simulink model "Dong_co_mot_chieu_KTSS"  (R2019a)
settings: Solver=VariableStepAuto  StartTime=0.0  StopTime=10.0  RelTol=1e-3
libraries: powerlib x5
settings Model: Creator=Admin  LastModifiedBy=Admin

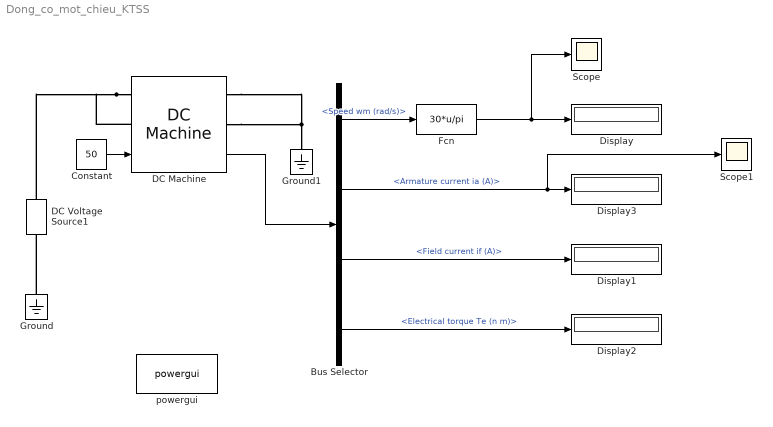
== system Dong_co_mot_chieu_KTSS ==
  Bus Selector : BusSelector  OutputSignals=Speed wm (rad/s),Armature current ia (A),Field current if (A),Electrical torque Te (n m)
  Constant : Constant  Value=50
  DC Machine : powerlib/Machines/DC Machine  PresetModel=No  MechanicalLoad=Torque TL  FieldType=Wound  ShowDetailedParameters=on  MeasurementBus=off  RLa="[ 0.2305  0.023]"  RLf="[ 298  59.6]"  Laf=1.247  MachineConstant=Torque constant (N.m/A)  Ke=1.8  Kt=1.8  J=0.28  Bm=0.000158  Tf=1.75  w0=1  Ifinit=1  TsPowergui=0  TsBlock=-1
      settings: SourceProductName=Simscape Electrical
  DC Voltage Source1 : powerlib/Electrical Sources/DC Voltage Source  Amplitude=120  Measurements=None
      settings: SourceProductName=Simscape Electrical
  Display{,1..3} (4 alike) : Display
  Fcn : Fcn  Expr=30*u/pi
  Ground : powerlib/Elements/Ground  LConnTagsString=a
      settings: SourceProductName=Simscape Electrical
  Ground1 : powerlib/Elements/Ground  LConnTagsString=a
      settings: SourceProductName=Simscape Electrical
  Scope : Scope
  Scope1 : Scope
  powergui : powerlib/powergui  Priority=1  SimulationMode=Continuous  SampleTime=50e-6  frequency=60  Iterations=50  frequencyindice=0  Pbase=100e6  ErrMax=1e-4  UnitsV=kV  UnitsW=MW  buscounter=0  FunctionMessages=off  echomessages=off  EnableUseOfTLC=off  CurrentSourceSwitches=off  DisableSnubberDevices=off  DisableRonSwitches=off  DisableVfSwitches=off  DisplayEquations=off  AutomaticDiscreteSolvers=off  SolverType=Tustin/Backward Euler (TBE)  Interpol=off  ExternalGateDelay=off  methode=off  Ts=100  x0status=blocks  SPID=on  SwTol=0  HookPort=off  NonlinearTolerance=0  nMaxIteration=15  ContinueOnMaxIteration=off  RestoreLinks=warning  ResistiveCurrentMeasurement=off  Frange=[0:2:500]  Ylog=off  Xlog=on  ShowGrid=off  save=off  variable=ZData  structure=0  ZoomFFT=off  StartTime=0.0  cycles=1  DisplayStyle=1  fundamental=60  FreqAxis=off  MaxFrequency=1000  frequencyindicesteady=1  RmsSteady=1  display=off
      settings: SourceProductName=Simscape Electrical
  wires:
  DC Machine/1 -> Bus Selector/1
  Bus Selector/1 -> Fcn/1  "<Speed wm (rad/s)>"
  Fcn/1 -> Scope/1, Display/1
  Bus Selector/2 -> Scope1/1, Display3/1  "<Armature current ia (A)>"
  Bus Selector/3 -> Display1/1  "<Field current if (A)>"
  Bus Selector/4 -> Display2/1  "<Electrical torque Te (n m)>"
  Constant/1 -> DC Machine/1
  connections:
  DC Machine/LConn2 -- DC Voltage Source1/RConn1 -- DC Machine/LConn1
  Ground/LConn1 -- DC Voltage Source1/LConn1
  DC Machine/RConn2 -- DC Machine/RConn1 -- Ground1/LConn1
